simulink model "speedloop"  (R2021b)
settings: Solver=FixedStepAuto  StartTime=0.0  StopTime=10.0  FixedStep=1e-4  RelTol=1e-3
values from neighbouring files (symbols this model uses):
  CurrKi = 0.17    [speedloop.sldd]
  CurrKp = 35.0    [speedloop.sldd]
  flux = 0.016884    [speedloop.sldd]
  Pn = 4.0    [speedloop.sldd]
  SpeedKi = 0.0144    [speedloop.sldd]
  SpeedKp = 0.03389    [speedloop.sldd]
  Ubus = 24.0    [speedloop.sldd]
undefined symbols (not defined in the file or in its folder): DiscIntNeverNeededParam, sigbuilder_block
libraries: slpidlib x3, mcbplantlib x1, autolibpmsmexterior x1
settings Model: DataDictionary=speedloop.sldd  Creator=ssc  LastModifiedBy=ssc

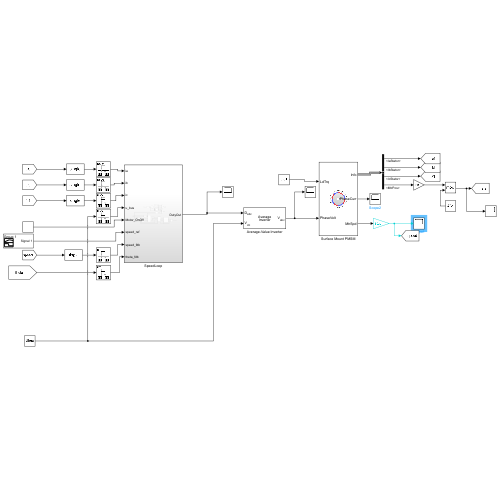
[thumbnail: Simulink's stored preview of the top-level diagram]
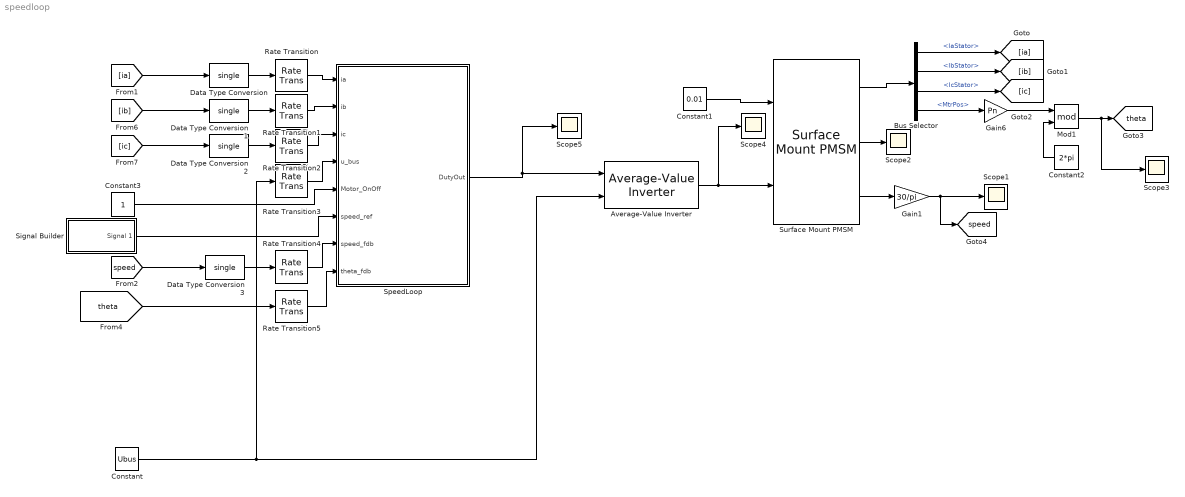
== system speedloop ==
  Average-Value Inverter : mcbplantlib/Average-Value Inverter
  Bus Selector : BusSelector  OutputSignals=IaStator,IbStator,IcStator,MtrPos
  Constant : Constant  Value=Ubus
  Constant1 : Constant  Value=0.01
  Constant2 : Constant  Value=2*pi  OutDataTypeStr=single
  Constant3 : Constant
  Data Type Conversion{,1..3} (4 alike) : DataTypeConversion  OutDataTypeStr=single
  Gain1 : Gain  Gain=30/pi  OutDataTypeStr=single
  Gain6 : Gain  Gain=Pn  OutDataTypeStr=single
  Mod1 : Math  Operator=mod  OutputSignalType=real  SaturateOnIntegerOverflow=on
  Rate Transition{,1..5} (6 alike) : RateTransition
  Scope{1..5} (5 alike) : Scope
  Signal Builder : Subsystem  Tag=STV Subsys  LoadFcn=sigbuilder_block('load');  StartFcn=sigbuilder_block('start');  StopFcn=sigbuilder_block('stop');  ClipboardFcn=sigbuilder_block('clipboard');  mask(Sigbuilder block){tuvar=[0:10]}
      mask help: Simulink:masks:SigbuilderBlock_MD
      mask init:
      | if ~strcmp(get_param(bdroot(gcbh),'SimulationStatus'),'stopped') tuvar = sigbuilder_block('maskInit'); end
      settings: CopyFcn=sigbuilder_block('copy');  DeleteFcn=sigbuilder_block('delete');  ModelCloseFcn=sigbuilder_block('modelClose');  PreSaveFcn=sigbuilder_block('preSave');  PauseFcn=sigbuilder_block('pause');  ContinueFcn=sigbuilder_block('continue');  NameChangeFcn=sigbuilder_block('namechange');  OpenFcn=sigbuilder_block('open',[367.2 103.2 550.8 400.2 ]);  CloseFcn=sigbuilder_block('close');
      mask Display: plot(0, 0, 100, 100,[2, 2, 32, 32, 2], [68, 8, 8, 68, 68],[32, 2], [38, 38], [32, 19, 2],[53, 60, 44], [32, 17, 17, 2],[16, 16, 31, 31]);txt = getActiveGroup(gcbh);text(2, 100, txt,'verticalAlignment', 'top');
  SpeedLoop : Subsystem
  Surface Mount PMSM : autolibpmsmexterior/Surface Mount PMSM  port_config=Torque  sim_type=Continuous  Ts=0.001  P=Pn  Rs=Rs  Ldq_=L  KConstText=Permanent flux linkage constant (lambda_pm):  lambda_pm=flux  Ke=159.9771  Kt=1.323  mechanical=[75e-6,8e-5,0]  idq0=[0 0]  theta_init=0  omega_init=0  KConst=flux  lambda_pm_calc=flux  RefBlkName='autolibpmsmexterior/Surface Mount PMSM'  aMode=5  Ldq="[0.0017      0.0017]"
      settings: SourceProductBaseCode=PW,DR,MT,UV,VE
  tag scope: speed=global, theta=global
  wires:
  SpeedLoop/1(DutyOut) -> Scope5/1, Average-Value Inverter/1
  Surface Mount PMSM/3 -> Gain1/1
  Surface Mount PMSM/1 -> Bus Selector/1
  Constant1/1 -> Surface Mount PMSM/1
  Bus Selector/1 -> [ia]  "<IaStator>"
  Gain1/1 -> Scope1/1, [speed]
  Surface Mount PMSM/2 -> Scope2/1
  Gain6/1 -> Mod1/1
  Bus Selector/2 -> [ib]  "<IbStator>"
  Mod1/1 -> Scope3/1, [theta]
  Constant2/1 -> Mod1/2
  Bus Selector/4 -> Gain6/1  "<MtrPos>"
  Constant/1 -> Rate Transition3/1, Average-Value Inverter/2
  Average-Value Inverter/1 -> Scope4/1, Surface Mount PMSM/2
  Bus Selector/3 -> [ic]  "<IcStator>"
  Data Type Conversion/1 -> Rate Transition/1
  Data Type Conversion1/1 -> Rate Transition1/1
  [ic] -> Data Type Conversion2/1
  [ib] -> Data Type Conversion1/1
  [ia] -> Data Type Conversion/1
  Data Type Conversion2/1 -> Rate Transition2/1
  Rate Transition/1 -> SpeedLoop/1(ia)
  Rate Transition1/1 -> SpeedLoop/2(ib)
  Rate Transition2/1 -> SpeedLoop/3(ic)
  Rate Transition3/1 -> SpeedLoop/4(u_bus)
  Constant3/1 -> SpeedLoop/5(Motor_OnOff)
  [speed] -> Data Type Conversion3/1
  Rate Transition4/1 -> SpeedLoop/7(speed_fdb)
  Data Type Conversion3/1 -> Rate Transition4/1
  Signal Builder/1(Signal 1) -> SpeedLoop/6(speed_ref)
  [theta] -> Rate Transition5/1
  Rate Transition5/1 -> SpeedLoop/8(theta_fdb)

== system speedloop/Signal Builder ==
  Demux : Demux  Tag=STV Demux  Outputs=1
      settings: DisplayOption=none
  FromWs : FromWorkspace  Tag=STV FromWs  VariableName=tuvar
      SigBuilderData=|
      | common.afterFinalStr = 'Extrapolate'
      | common.sampleTime = 0
      | dataSet.timeRange = [0 10]
      | dataSet.name = 'Group 1'
      | sbobj.Groups.Name = 'Group 1'
      | sbobj.Groups.Signals.Name = 'Signal 1'
      | sbobj.Groups.Signals.XData = [0 4 4 6 6 10]
      | sbobj.Groups.Signals.YData = [800 800 1000 1000 1200 1200]
  Signal 1 : Outport  Tag=STV Outport
  wires:
  Demux/1 -> Signal 1/1
  FromWs/1 -> Demux/1

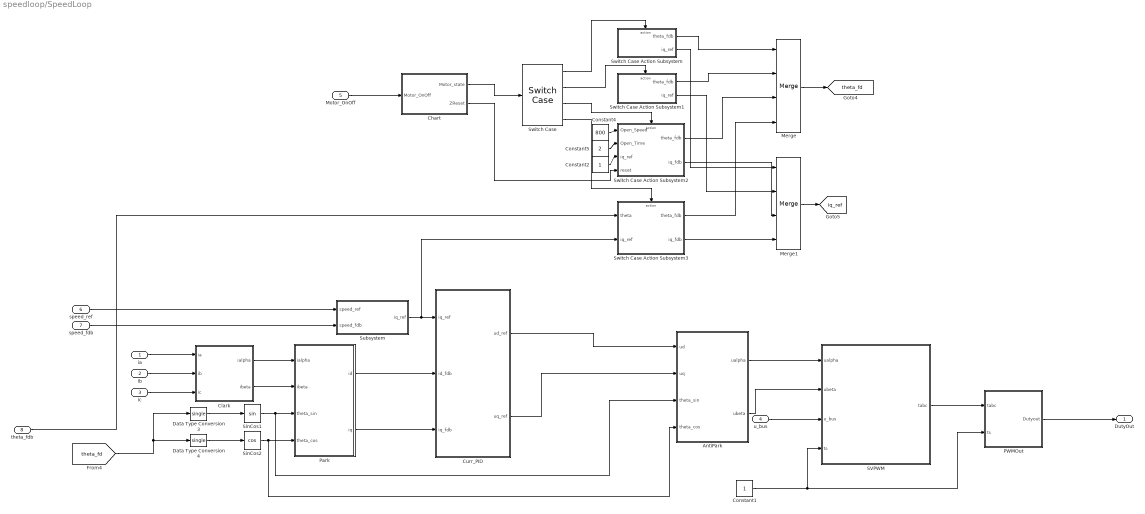
== system speedloop/SpeedLoop ==
  ia : Inport
  ib : Inport  Port=2
  ic : Inport  Port=3
  u_bus : Inport  Port=4
  Motor_OnOff : Inport  Port=5
  speed_ref : Inport  Port=6
  speed_fdb : Inport  Port=7
  theta_fdb : Inport  Port=8
  AntiPark : Subsystem
  Chart : Stateflow chart  TreatAsAtomicUnit=on
  Clark : Subsystem
  Constant1 : Constant
  Constant2 : Constant
  Constant4 : Constant  Value=800
  Constant5 : Constant  Value=2
  Curr_PID : Subsystem
  Data Type Conversion3 : DataTypeConversion  OutDataTypeStr=single
  Data Type Conversion4 : DataTypeConversion  OutDataTypeStr=single
  Merge : Merge  Inputs=4
  Merge1 : Merge  Inputs=4
  PWMOut : Subsystem
  Park : Subsystem
  SVPWM : Subsystem
  SinCos1 : Trigonometry
  SinCos2 : Trigonometry  Operator=cos
  Subsystem : Subsystem
  Switch Case : SwitchCase  CaseConditions={1,2,3,4}  ShowDefaultCase=off
  Switch Case Action Subsystem : Subsystem  TreatAsAtomicUnit=on
  Switch Case Action Subsystem1 : Subsystem  TreatAsAtomicUnit=on
  Switch Case Action Subsystem2 : Subsystem  TreatAsAtomicUnit=on
  Switch Case Action Subsystem3 : Subsystem  TreatAsAtomicUnit=on
  DutyOut : Outport
  tag scope: iq_ref=global, theta_fd=global
  wires:
  SinCos1/1 -> AntiPark/3(theta_sin), Park/3(theta_sin)
  Constant1/1 -> PWMOut/2(ts), SVPWM/4(ts)
  Switch Case Action Subsystem2/2(iq_fdb) -> Merge1/3
  Park/2(iq) -> Curr_PID/3(iq_fdb)
  Merge1/1 -> [iq_ref]
  Switch Case Action Subsystem/1(theta_fdb) -> Merge/1
  Switch Case Action Subsystem3/2(iq_fdb) -> Merge1/4
  Constant5/1 -> Switch Case Action Subsystem2/2(Open_Time)
  PWMOut/1(Dutyout) -> DutyOut/1
  SVPWM/1(tabc) -> PWMOut/1(tabc)
  Merge/1 -> [theta_fd]
  AntiPark/2(ubeta) -> SVPWM/2(ubeta)
  Chart/1(Motor_state) -> Switch Case/1
  ia/1 -> Clark/1(ia)
  Switch Case/4 -> Switch Case Action Subsystem3/Action
  theta_fdb/1 -> Switch Case Action Subsystem3/1(theta)
  Constant4/1 -> Switch Case Action Subsystem2/1(Open_Speed)
  Curr_PID/2(uq_ref) -> AntiPark/2(uq)
  Data Type Conversion3/1 -> SinCos1/1
  Switch Case Action Subsystem2/1(theta_fdb) -> Merge/3
  Switch Case Action Subsystem1/1(theta_fdb) -> Merge/2
  Clark/2(ibeta) -> Park/2(ibeta)
  Switch Case Action Subsystem1/2(iq_ref) -> Merge1/2
  u_bus/1 -> SVPWM/3(u_bus)
  Clark/1(ialpha) -> Park/1(ialpha)
  SinCos2/1 -> AntiPark/4(theta_cos), Park/4(theta_cos)
  Switch Case/1 -> Switch Case Action Subsystem/Action
  AntiPark/1(ualpha) -> SVPWM/1(ualpha)
  Switch Case/3 -> Switch Case Action Subsystem2/Action
  Park/1(id) -> Curr_PID/2(id_fdb)
  Switch Case/2 -> Switch Case Action Subsystem1/Action
  Data Type Conversion4/1 -> SinCos2/1
  ib/1 -> Clark/2(ib)
  Switch Case Action Subsystem/2(iq_ref) -> Merge1/1
  Curr_PID/1(ud_ref) -> AntiPark/1(ud)
  ic/1 -> Clark/3(ic)
  Motor_OnOff/1 -> Chart/1(Motor_OnOff)
  speed_ref/1 -> Subsystem/1(speed_ref)
  speed_fdb/1 -> Subsystem/2(speed_fdb)
  Constant2/1 -> Switch Case Action Subsystem2/3(iq_ref)
  Chart/2(ZReset) -> Switch Case Action Subsystem2/4(reset)
  [theta_fd] -> Data Type Conversion4/1, Data Type Conversion3/1
  Subsystem/1(iq_ref) -> Switch Case Action Subsystem3/2(iq_ref), Curr_PID/1(iq_ref)
  Switch Case Action Subsystem3/1(theta_fdb) -> Merge/4

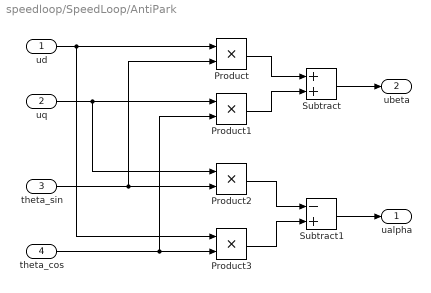
== system speedloop/SpeedLoop/AntiPark ==
  ud : Inport
  uq : Inport  Port=2
  theta_sin : Inport  Port=3
  theta_cos : Inport  Port=4
  Product{,1..3} (4 alike) : Product
  Subtract : Sum
  Subtract1 : Sum  Inputs=-+
  ualpha : Outport
  ubeta : Outport  Port=2
  wires:
  ud/1 -> Product/1, Product3/1
  theta_sin/1 -> Product2/2, Product/2
  uq/1 -> Product1/1, Product2/1
  theta_cos/1 -> Product3/2, Product1/2
  Product/1 -> Subtract/1
  Product1/1 -> Subtract/2
  Product2/1 -> Subtract1/1
  Product3/1 -> Subtract1/2
  Subtract/1 -> ubeta/1
  Subtract1/1 -> ualpha/1

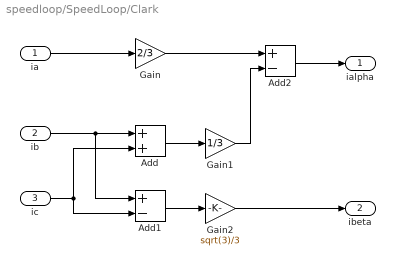
== system speedloop/SpeedLoop/Clark ==
  ia : Inport
  ib : Inport  Port=2
  ic : Inport  Port=3
  Add : Sum
  Add1 : Sum  Inputs=+-
  Add2 : Sum  Inputs=+-
  Gain : Gain  Gain=2/3
  Gain1 : Gain  Gain=1/3
  Gain2 : Gain  Gain=sqrt(3)/3
  ialpha : Outport
  ibeta : Outport  Port=2
  wires:
  ia/1 -> Gain/1
  ib/1 -> Add1/1, Add/1
  ic/1 -> Add1/2, Add/2
  Add/1 -> Gain1/1
  Add1/1 -> Gain2/1
  Gain1/1 -> Add2/2
  Gain/1 -> Add2/1
  Gain2/1 -> ibeta/1
  Add2/1 -> ialpha/1

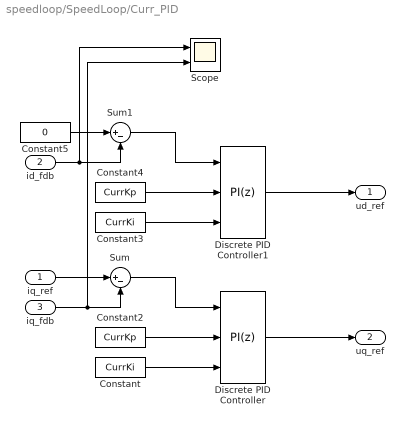
== system speedloop/SpeedLoop/Curr_PID ==
  iq_ref : Inport
  id_fdb : Inport  Port=2
  iq_fdb : Inport  Port=3
  Constant : Constant  Value=CurrKi
  Constant2 : Constant  Value=CurrKp
  Constant3 : Constant  Value=CurrKi
  Constant4 : Constant  Value=CurrKp
  Constant5 : Constant  Value=0
  Discrete PID Controller : slpidlib/PID Controller  Controller=PI  Form=Parallel  TimeDomain=Discrete-time  UseExternalTs=off  SampleTime=-1  IntegratorMethod=Forward Euler  FilterMethod=Forward Euler  ControllerParametersSource=external  P=1  I=1  D=0  UseFilter=on  N=100  TunerSelectOption=Transfer Function Based (PID Tuner App)  InitialConditionSource=internal  InitialConditionForIntegrator=0  InitialConditionForFilter=0  DifferentiatorICPrevScaledInput=0  ExternalReset=none  TrackingMode=off  Kt=1  LimitOutput=on  SatLimitsSource=internal  UpperSaturationLimit=Ubus/sqrt(3)  LowerSaturationLimit=-Ubus/sqrt(3)  LinearizeAsGain=off  AntiWindupMode=clamping  Kb=1  POutMin=[]  POutMax=[]  IOutMin=[]  IOutMax=[]  DOutMin=[]  DOutMax=[]  NOutMin=[]  NOutMax=[]  SumOutMin=[]  SumOutMax=[]  SaturationOutMin=[]  SaturationOutMax=[]  PParamMin=[]  PParamMax=[]  IParamMin=[]  IParamMax=[]  DParamMin=[]  DParamMax=[]  NParamMin=[]  NParamMax=[]  KbParamMin=[]  KbParamMax=[]  KtParamMin=[]  KtParamMax=[]  KbOutMin=[]  KbOutMax=[]  KtOutMin=[]  KtOutMax=[]  IntegratorOutMin=[]  IntegratorOutMax=[]  FilterOutMin=[]  FilterOutMax=[]  SumI1OutMin=[]  SumI1OutMax=[]  SumI2OutMin=[]  SumI2OutMax=[]  SumI3OutMin=[]  SumI3OutMax=[]  SumI4OutMin=[]  SumI4OutMax=[]  SumDOutMin=[]  SumDOutMax=[]  DifferentiatorOutMin=[]  DifferentiatorOutMax=[]  FilterDiffOutCoefMin=[]  FilterDiffOutCoefMax=[]  ReciprocalOutMin=[]  ReciprocalOutMax=[]  SumDenOutMin=[]  SumDenOutMax=[]  SumNumOutMin=[]  SumNumOutMax=[]  DivideOutMin=[]  DivideOutMax=[]  UdiffTsProdOutMin=[]  UdiffTsProdOutMax=[]  NTsProdOutMin=[]  NTsProdOutMax=[]  UintegralTsProdOutMin=[]  UintegralTsProdOutMax=[]  UngainTsProdOutMin=[]  UngainTsProdOutMax=[]  IntegratorContinuousStateAttributes=''  IntegratorStateMustResolveToSignalObject=off  IntegratorRTWStateStorageClass=Auto  FilterContinuousStateAttributes=''  FilterStateMustResolveToSignalObject=off  FilterRTWStateStorageClass=Auto  ParallelPVariant=ExternalParameters  IdealPVariant=Disabled  IVariant=ExternalParameters  DVariant=Disabled  IntegratorVariant=Discrete  SatVariant=Enabled  AWVariant=DiscClampingParallel  PCopyVariant=Disabled  TRVariant=Disabled  FdbkBlocksVariant=Forward  IdealPFdbkVariant=Disabled  SatFdbkVariant=Disabled  DerivativeFilterVariant=Disabled  NVariant=Disabled  NCopyVariant=Disabled_SignalSpec  FilterICVariant=Disabled  IntegratorICVariant=InternalICs  ExternalResetVariant=Disabled  TRSumVariant=Passthrough  SumFdbkVariant=Disabled  SumVariant=Sum_PI  TsampFilterVariant=InternalTs  TsampNgainVariant=Passthrough  TsampIntegralVariant=Passthrough  ExternalSaturationOutDataTypeStr=Inherit: Same as second input
  Discrete PID Controller1 : slpidlib/PID Controller  Controller=PI  Form=Parallel  TimeDomain=Discrete-time  UseExternalTs=off  SampleTime=-1  IntegratorMethod=Forward Euler  FilterMethod=Forward Euler  ControllerParametersSource=external  P=1  I=1  D=0  UseFilter=on  N=100  TunerSelectOption=Transfer Function Based (PID Tuner App)  InitialConditionSource=internal  InitialConditionForIntegrator=0  InitialConditionForFilter=0  DifferentiatorICPrevScaledInput=0  ExternalReset=none  TrackingMode=off  Kt=1  LimitOutput=on  SatLimitsSource=internal  UpperSaturationLimit=Ubus/sqrt(3)  LowerSaturationLimit=-Ubus/sqrt(3)  LinearizeAsGain=off  AntiWindupMode=clamping  Kb=1  POutMin=[]  POutMax=[]  IOutMin=[]  IOutMax=[]  DOutMin=[]  DOutMax=[]  NOutMin=[]  NOutMax=[]  SumOutMin=[]  SumOutMax=[]  SaturationOutMin=[]  SaturationOutMax=[]  PParamMin=[]  PParamMax=[]  IParamMin=[]  IParamMax=[]  DParamMin=[]  DParamMax=[]  NParamMin=[]  NParamMax=[]  KbParamMin=[]  KbParamMax=[]  KtParamMin=[]  KtParamMax=[]  KbOutMin=[]  KbOutMax=[]  KtOutMin=[]  KtOutMax=[]  IntegratorOutMin=[]  IntegratorOutMax=[]  FilterOutMin=[]  FilterOutMax=[]  SumI1OutMin=[]  SumI1OutMax=[]  SumI2OutMin=[]  SumI2OutMax=[]  SumI3OutMin=[]  SumI3OutMax=[]  SumI4OutMin=[]  SumI4OutMax=[]  SumDOutMin=[]  SumDOutMax=[]  DifferentiatorOutMin=[]  DifferentiatorOutMax=[]  FilterDiffOutCoefMin=[]  FilterDiffOutCoefMax=[]  ReciprocalOutMin=[]  ReciprocalOutMax=[]  SumDenOutMin=[]  SumDenOutMax=[]  SumNumOutMin=[]  SumNumOutMax=[]  DivideOutMin=[]  DivideOutMax=[]  UdiffTsProdOutMin=[]  UdiffTsProdOutMax=[]  NTsProdOutMin=[]  NTsProdOutMax=[]  UintegralTsProdOutMin=[]  UintegralTsProdOutMax=[]  UngainTsProdOutMin=[]  UngainTsProdOutMax=[]  IntegratorContinuousStateAttributes=''  IntegratorStateMustResolveToSignalObject=off  IntegratorRTWStateStorageClass=Auto  FilterContinuousStateAttributes=''  FilterStateMustResolveToSignalObject=off  FilterRTWStateStorageClass=Auto  ParallelPVariant=ExternalParameters  IdealPVariant=Disabled  IVariant=ExternalParameters  DVariant=Disabled  IntegratorVariant=Discrete  SatVariant=Enabled  AWVariant=DiscClampingParallel  PCopyVariant=Disabled  TRVariant=Disabled  FdbkBlocksVariant=Forward  IdealPFdbkVariant=Disabled  SatFdbkVariant=Disabled  DerivativeFilterVariant=Disabled  NVariant=Disabled  NCopyVariant=Disabled_SignalSpec  FilterICVariant=Disabled  IntegratorICVariant=InternalICs  ExternalResetVariant=Disabled  TRSumVariant=Passthrough  SumFdbkVariant=Disabled  SumVariant=Sum_PI  TsampFilterVariant=InternalTs  TsampNgainVariant=Passthrough  TsampIntegralVariant=Passthrough  ExternalSaturationOutDataTypeStr=Inherit: Same as second input
  Scope : Scope  NumInputPorts=2
  Sum : Sum  Inputs=|+-
  Sum1 : Sum  Inputs=|+-
  ud_ref : Outport
  uq_ref : Outport  Port=2
  wires:
  Constant2/1 -> Discrete PID Controller/2
  Constant3/1 -> Discrete PID Controller1/3
  Sum1/1 -> Discrete PID Controller1/1
  Sum/1 -> Discrete PID Controller/1
  Constant/1 -> Discrete PID Controller/3
  iq_ref/1 -> Sum/1
  Discrete PID Controller/1 -> uq_ref/1
  Constant4/1 -> Discrete PID Controller1/2
  Discrete PID Controller1/1 -> ud_ref/1
  Constant5/1 -> Sum1/1
  iq_fdb/1 -> Scope/2, Sum/2
  id_fdb/1 -> Scope/1, Sum1/2

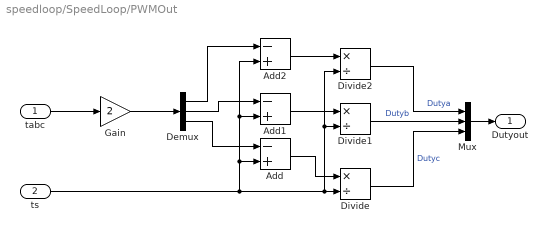
== system speedloop/SpeedLoop/PWMOut ==
  tabc : Inport
  ts : Inport  Port=2
  Add : Sum  Inputs=-+
  Add1 : Sum  Inputs=-+
  Add2 : Sum  Inputs=-+
  Demux : Demux  Outputs=3
  Divide : Product  Inputs=*/
  Divide1 : Product  Inputs=*/
  Divide2 : Product  Inputs=*/
  Gain : Gain  Gain=2
  Mux : Mux  Inputs=3
  Dutyout : Outport
  wires:
  tabc/1 -> Gain/1
  Gain/1 -> Demux/1
  ts/1 -> Add1/2, Add2/2, Add/2, Divide2/2, Divide1/2, Divide/2
  Demux/3 -> Add/1
  Add/1 -> Divide/1
  Divide/1 -> Mux/3  "Dutyc"
  Demux/1 -> Add2/1
  Add1/1 -> Divide1/1
  Add2/1 -> Divide2/1
  Demux/2 -> Add1/1
  Divide1/1 -> Mux/2  "Dutyb"
  Divide2/1 -> Mux/1  "Dutya"
  Mux/1 -> Dutyout/1

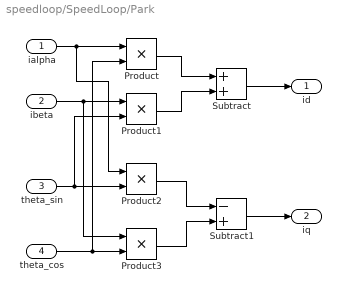
== system speedloop/SpeedLoop/Park ==
  ialpha : Inport
  ibeta : Inport  Port=2
  theta_sin : Inport  Port=3
  theta_cos : Inport  Port=4
  Product{,1..3} (4 alike) : Product
  Subtract : Sum
  Subtract1 : Sum  Inputs=-+
  id : Outport
  iq : Outport  Port=2
  wires:
  ialpha/1 -> Product2/1, Product/1
  theta_cos/1 -> Product/2, Product3/2
  ibeta/1 -> Product3/1, Product1/1
  theta_sin/1 -> Product1/2, Product2/2
  Product/1 -> Subtract/1
  Product1/1 -> Subtract/2
  Subtract/1 -> id/1
  Product2/1 -> Subtract1/1
  Product3/1 -> Subtract1/2
  Subtract1/1 -> iq/1

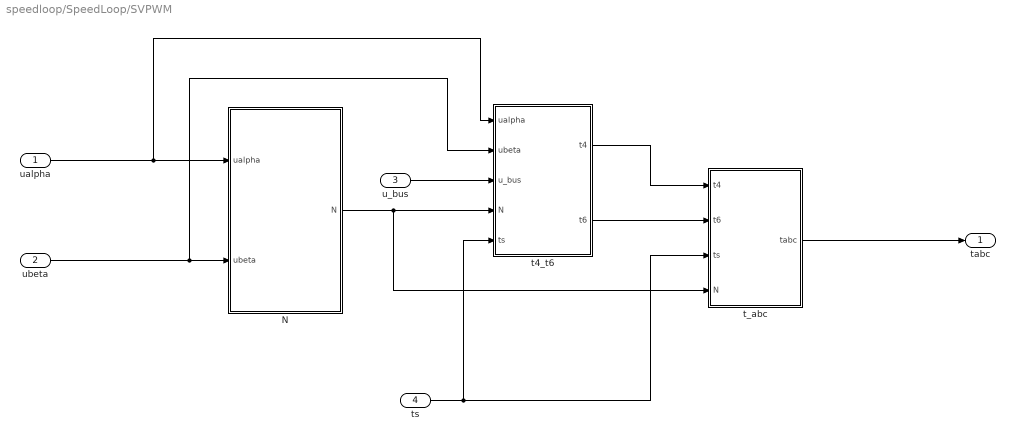
== system speedloop/SpeedLoop/SVPWM ==
  ualpha : Inport
  ubeta : Inport  Port=2
  u_bus : Inport  Port=3
  ts : Inport  Port=4
  N : Subsystem
  t4_t6 : Subsystem
  t_abc : Subsystem
  tabc : Outport
  wires:
  ubeta/1 -> t4_t6/2(ubeta), N/2(ubeta)
  t4_t6/1(t4) -> t_abc/1(t4)
  N/1(N) -> t_abc/4(N), t4_t6/4(N)
  ualpha/1 -> t4_t6/1(ualpha), N/1(ualpha)
  t4_t6/2(t6) -> t_abc/2(t6)
  u_bus/1 -> t4_t6/3(u_bus)
  ts/1 -> t_abc/3(ts), t4_t6/5(ts)
  t_abc/1(tabc) -> tabc/1

== system speedloop/SpeedLoop/Subsystem ==
  speed_ref : Inport
  speed_fdb : Inport  Port=2
  Constant2 : Constant  Value=SpeedKp
  Constant3 : Constant  Value=SpeedKi
  Discrete PID Controller1 : slpidlib/PID Controller  Controller=PI  Form=Parallel  TimeDomain=Discrete-time  UseExternalTs=off  SampleTime=-1  IntegratorMethod=Forward Euler  FilterMethod=Forward Euler  ControllerParametersSource=external  P=1  I=1  D=0  UseFilter=on  N=100  TunerSelectOption=Transfer Function Based (PID Tuner App)  InitialConditionSource=internal  InitialConditionForIntegrator=0  InitialConditionForFilter=0  DifferentiatorICPrevScaledInput=0  ExternalReset=none  TrackingMode=off  Kt=1  LimitOutput=on  SatLimitsSource=internal  UpperSaturationLimit=3  LowerSaturationLimit=-3  LinearizeAsGain=off  AntiWindupMode=clamping  Kb=1  POutMin=[]  POutMax=[]  IOutMin=[]  IOutMax=[]  DOutMin=[]  DOutMax=[]  NOutMin=[]  NOutMax=[]  SumOutMin=[]  SumOutMax=[]  SaturationOutMin=[]  SaturationOutMax=[]  PParamMin=[]  PParamMax=[]  IParamMin=[]  IParamMax=[]  DParamMin=[]  DParamMax=[]  NParamMin=[]  NParamMax=[]  KbParamMin=[]  KbParamMax=[]  KtParamMin=[]  KtParamMax=[]  KbOutMin=[]  KbOutMax=[]  KtOutMin=[]  KtOutMax=[]  IntegratorOutMin=[]  IntegratorOutMax=[]  FilterOutMin=[]  FilterOutMax=[]  SumI1OutMin=[]  SumI1OutMax=[]  SumI2OutMin=[]  SumI2OutMax=[]  SumI3OutMin=[]  SumI3OutMax=[]  SumI4OutMin=[]  SumI4OutMax=[]  SumDOutMin=[]  SumDOutMax=[]  DifferentiatorOutMin=[]  DifferentiatorOutMax=[]  FilterDiffOutCoefMin=[]  FilterDiffOutCoefMax=[]  ReciprocalOutMin=[]  ReciprocalOutMax=[]  SumDenOutMin=[]  SumDenOutMax=[]  SumNumOutMin=[]  SumNumOutMax=[]  DivideOutMin=[]  DivideOutMax=[]  UdiffTsProdOutMin=[]  UdiffTsProdOutMax=[]  NTsProdOutMin=[]  NTsProdOutMax=[]  UintegralTsProdOutMin=[]  UintegralTsProdOutMax=[]  UngainTsProdOutMin=[]  UngainTsProdOutMax=[]  IntegratorContinuousStateAttributes=''  IntegratorStateMustResolveToSignalObject=off  IntegratorRTWStateStorageClass=Auto  FilterContinuousStateAttributes=''  FilterStateMustResolveToSignalObject=off  FilterRTWStateStorageClass=Auto  ParallelPVariant=ExternalParameters  IdealPVariant=Disabled  IVariant=ExternalParameters  DVariant=Disabled  IntegratorVariant=Discrete  SatVariant=Enabled  AWVariant=DiscClampingParallel  PCopyVariant=Disabled  TRVariant=Disabled  FdbkBlocksVariant=Forward  IdealPFdbkVariant=Disabled  SatFdbkVariant=Disabled  DerivativeFilterVariant=Disabled  NVariant=Disabled  NCopyVariant=Disabled_SignalSpec  FilterICVariant=Disabled  IntegratorICVariant=InternalICs  ExternalResetVariant=Disabled  TRSumVariant=Passthrough  SumFdbkVariant=Disabled  SumVariant=Sum_PI  TsampFilterVariant=InternalTs  TsampNgainVariant=Passthrough  TsampIntegralVariant=Passthrough  ExternalSaturationOutDataTypeStr=Inherit: Same as second input
  Sum1 : Sum  Inputs=|+-
  iq_ref : Outport
  wires:
  speed_fdb/1 -> Sum1/2
  Constant2/1 -> Discrete PID Controller1/2
  speed_ref/1 -> Sum1/1
  Discrete PID Controller1/1 -> iq_ref/1
  Sum1/1 -> Discrete PID Controller1/1
  Constant3/1 -> Discrete PID Controller1/3

== system speedloop/SpeedLoop/Switch Case Action Subsystem ==
  Action Port : ActionPort  ActionPortLabel=case [ 1 ]:
  Constant : Constant  Value=0
  Constant1 : Constant  Value=0
  theta_fdb : Outport
  iq_ref : Outport  Port=2
  wires:
  Constant/1 -> theta_fdb/1
  Constant1/1 -> iq_ref/1

== system speedloop/SpeedLoop/Switch Case Action Subsystem1 ==
  Action Port : ActionPort  ActionPortLabel=case [ 2 ]:
  Constant : Constant  Value=0
  Constant1 : Constant
  theta_fdb : Outport
  iq_ref : Outport  Port=2
  wires:
  Constant/1 -> theta_fdb/1
  Constant1/1 -> iq_ref/1

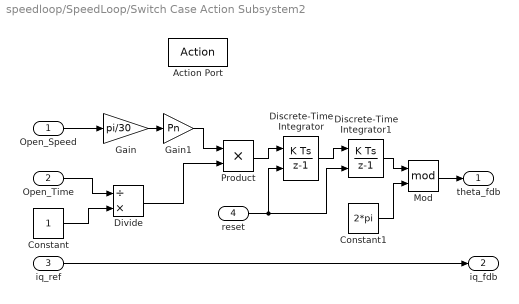
== system speedloop/SpeedLoop/Switch Case Action Subsystem2 ==
  Open_Speed : Inport
  Open_Time : Inport  Port=2
  iq_ref : Inport  Port=3
  reset : Inport  Port=4
  Action Port : ActionPort  ActionPortLabel=case [ 3 ]:
  Constant : Constant
  Constant1 : Constant  Value=2*pi  OutDataTypeStr=double
  Discrete-Time Integrator : DiscreteIntegrator  ExternalReset=rising  SampleTime=-1  ICPrevOutput=DiscIntNeverNeededParam  ICPrevScaledInput=DiscIntNeverNeededParam
  Discrete-Time Integrator1 : DiscreteIntegrator  ExternalReset=rising  SampleTime=-1  ICPrevOutput=DiscIntNeverNeededParam  ICPrevScaledInput=DiscIntNeverNeededParam
  Divide : Product  Inputs=/*
  Gain : Gain  Gain=pi/30
  Gain1 : Gain  Gain=Pn
  Mod : Math  Operator=mod  SaturateOnIntegerOverflow=on
  Product : Product
  theta_fdb : Outport
  iq_fdb : Outport  Port=2
  wires:
  Open_Speed/1 -> Gain/1
  Gain/1 -> Gain1/1
  Gain1/1 -> Product/1
  Open_Time/1 -> Divide/1
  Constant/1 -> Divide/2
  Divide/1 -> Product/2
  Product/1 -> Discrete-Time Integrator/1
  iq_ref/1 -> iq_fdb/1
  Discrete-Time Integrator/1 -> Discrete-Time Integrator1/1
  Mod/1 -> theta_fdb/1
  Constant1/1 -> Mod/2
  Discrete-Time Integrator1/1 -> Mod/1
  reset/1 -> Discrete-Time Integrator/2, Discrete-Time Integrator1/2

== system speedloop/SpeedLoop/Switch Case Action Subsystem3 ==
  theta : Inport
  iq_ref : Inport  Port=2
  Action Port : ActionPort  ActionPortLabel=case [ 4 ]:
  Data Type Conversion1 : DataTypeConversion  OutDataTypeStr=double
  theta_fdb : Outport
  iq_fdb : Outport  Port=2
  wires:
  iq_ref/1 -> iq_fdb/1
  theta/1 -> Data Type Conversion1/1
  Data Type Conversion1/1 -> theta_fdb/1

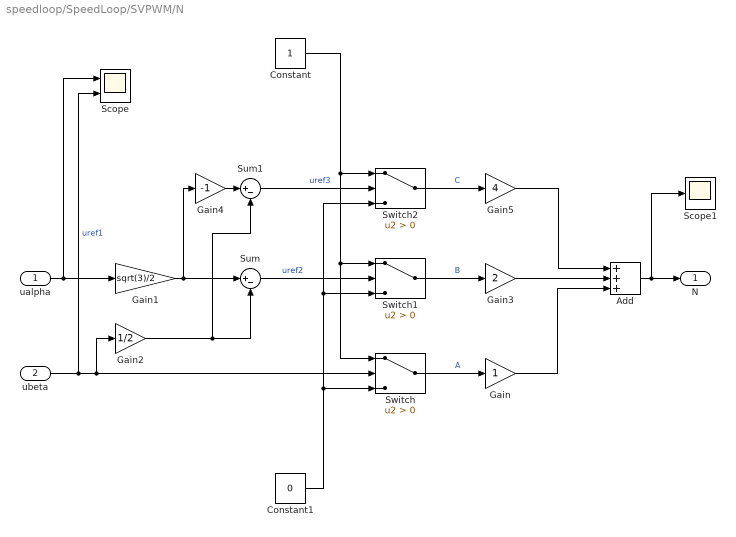
== system speedloop/SpeedLoop/SVPWM/N ==
  ualpha : Inport
  ubeta : Inport  Port=2
  Add : Sum  Inputs=+++
  Constant : Constant  OutDataTypeStr=single
  Constant1 : Constant  Value=0  OutDataTypeStr=single
  Gain : Gain
  Gain1 : Gain  Gain=sqrt(3)/2
  Gain2 : Gain  Gain=1/2
  Gain3 : Gain  Gain=2
  Gain4 : Gain  Gain=-1
  Gain5 : Gain  Gain=4
  Scope : Scope  NumInputPorts=2
  Scope1 : Scope
  Sum : Sum  Inputs=|+-
  Sum1 : Sum  Inputs=|+-
  Switch : Switch  Criteria=u2 > Threshold
  Switch1 : Switch  Criteria=u2 > Threshold
  Switch2 : Switch  Criteria=u2 > Threshold
  N : Outport
  wires:
  ualpha/1 -> Gain1/1, Scope/1
  ubeta/1 -> Switch/2, Gain2/1, Scope/2  "uref1"
  Constant/1 -> Switch2/1, Switch1/1, Switch/1
  Constant1/1 -> Switch2/3, Switch1/3, Switch/3
  Switch/1 -> Gain/1  "A"
  Gain1/1 -> Gain4/1, Sum/1
  Gain2/1 -> Sum1/2, Sum/2
  Sum/1 -> Switch1/2  "uref2"
  Switch1/1 -> Gain3/1  "B"
  Gain4/1 -> Sum1/1
  Sum1/1 -> Switch2/2  "uref3"
  Switch2/1 -> Gain5/1  "C"
  Gain3/1 -> Add/2
  Add/1 -> Scope1/1, N/1
  Gain/1 -> Add/3
  Gain5/1 -> Add/1

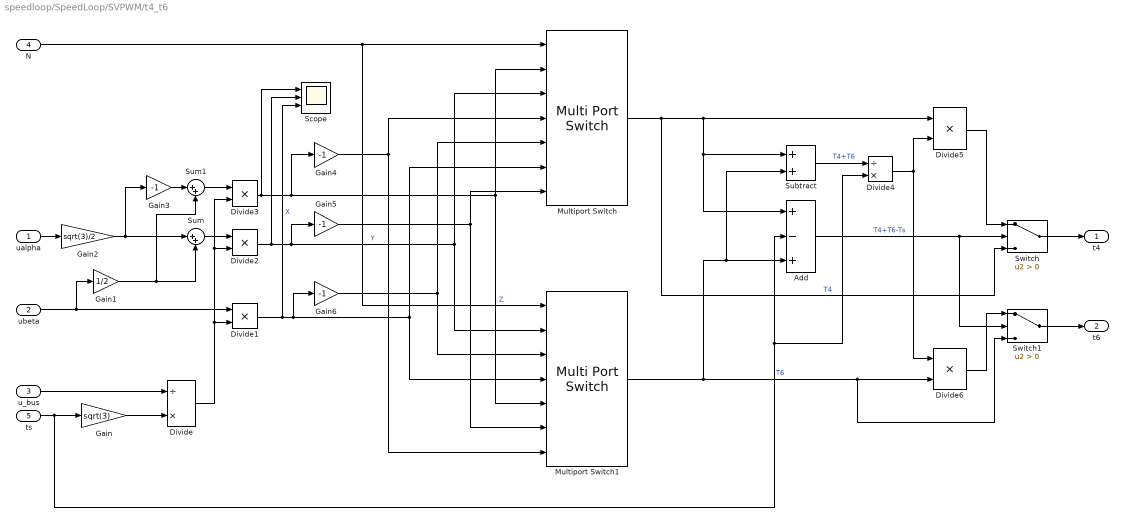
== system speedloop/SpeedLoop/SVPWM/t4_t6 ==
  ualpha : Inport
  ubeta : Inport  Port=2
  u_bus : Inport  Port=3
  N : Inport  Port=4
  ts : Inport  Port=5
  Add : Sum  Inputs=+-+
  Divide : Product  Inputs=/*
  Divide{1..3,5..6} (5 alike) : Product  Inputs=**
  Divide4 : Product  Inputs=/*
  Gain : Gain  Gain=sqrt(3)
  Gain1 : Gain  Gain=1/2
  Gain2 : Gain  Gain=sqrt(3)/2
  Gain{3..6} (4 alike) : Gain  Gain=-1
  Multiport Switch : MultiPortSwitch  Inputs=6  DiagnosticForDefault=None
  Multiport Switch1 : MultiPortSwitch  Inputs=6  DiagnosticForDefault=None
  Scope : Scope  NumInputPorts=3
  Subtract : Sum
  Sum : Sum  Inputs=|++
  Sum1 : Sum  Inputs=|++
  Switch : Switch  Criteria=u2 > Threshold
  Switch1 : Switch  Criteria=u2 > Threshold
  t4 : Outport
  t6 : Outport  Port=2
  wires:
  ts/1 -> Gain/1, Divide4/2, Add/2
  u_bus/1 -> Divide/1
  Gain/1 -> Divide/2
  ubeta/1 -> Gain1/1, Divide1/1
  Divide/1 -> Divide3/2, Divide2/2, Divide1/2
  Divide1/1 -> Scope/3, Multiport Switch1/4, Multiport Switch/6, Gain6/1  "X"
  ualpha/1 -> Gain2/1
  Gain1/1 -> Sum1/2, Sum/2
  Gain2/1 -> Gain3/1, Sum/1
  Sum/1 -> Divide2/1
  Divide2/1 -> Scope/2, Multiport Switch1/2, Multiport Switch/3, Gain5/1  "Y"
  Gain3/1 -> Sum1/1
  Sum1/1 -> Divide3/1
  Divide3/1 -> Scope/1, Gain4/1, Multiport Switch1/5, Multiport Switch/2  "Z"
  N/1 -> Multiport Switch1/1, Multiport Switch/1
  Multiport Switch/1 -> Switch/3, Divide5/1, Subtract/1, Add/1  "T4"
  Gain6/1 -> Multiport Switch1/3, Multiport Switch/5
  Gain4/1 -> Multiport Switch1/7, Multiport Switch/4
  Gain5/1 -> Multiport Switch1/6, Multiport Switch/7
  Add/1 -> Switch1/2, Switch/2  "T4+T6-Ts"
  Multiport Switch1/1 -> Switch1/3, Divide6/2, Subtract/2, Add/3  "T6"
  Subtract/1 -> Divide4/1  "T4+T6"
  Divide4/1 -> Divide5/2, Divide6/1
  Divide5/1 -> Switch/1
  Divide6/1 -> Switch1/1
  Switch/1 -> t4/1
  Switch1/1 -> t6/1

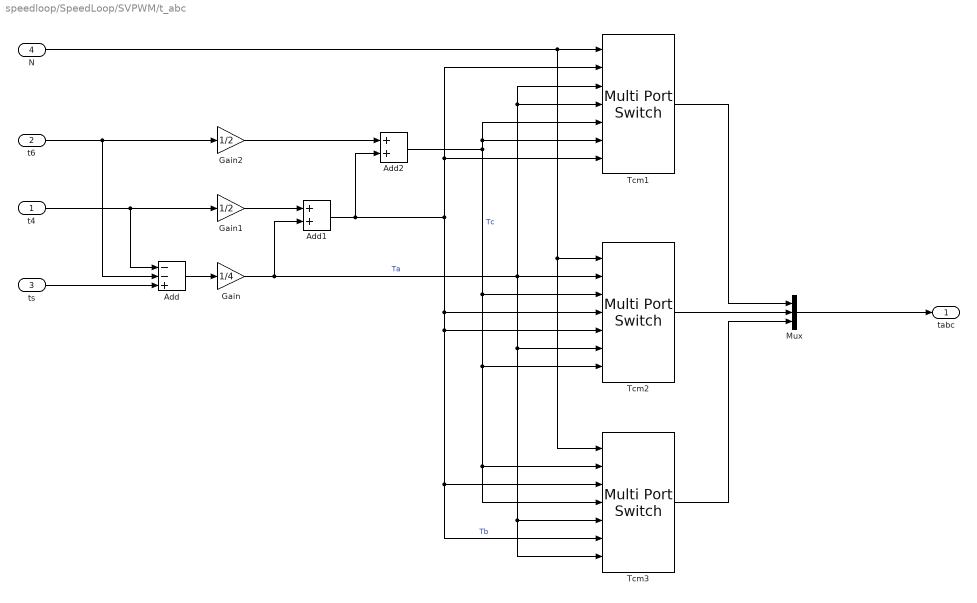
== system speedloop/SpeedLoop/SVPWM/t_abc ==
  t4 : Inport
  t6 : Inport  Port=2
  ts : Inport  Port=3
  N : Inport  Port=4
  Add : Sum  Inputs=--+
  Add1 : Sum
  Add2 : Sum
  Gain : Gain  Gain=1/4
  Gain1 : Gain  Gain=1/2
  Gain2 : Gain  Gain=1/2
  Mux : Mux  Inputs=3
  "Tcm1 " : MultiPortSwitch  Inputs=6  DiagnosticForDefault=None
  Tcm2 : MultiPortSwitch  Inputs=6  DiagnosticForDefault=None
  Tcm3 : MultiPortSwitch  Inputs=6  DiagnosticForDefault=None
  tabc : Outport
  wires:
  ts/1 -> Add/3
  t6/1 -> Add/2, Gain2/1
  t4/1 -> Add/1, Gain1/1
  Add/1 -> Gain/1
  Gain/1 -> Tcm2/6, Tcm3/7, Tcm3/5, "Tcm1 "/4, "Tcm1 "/3, Tcm2/2, Add1/2  "Ta"
  Gain1/1 -> Add1/1
  Gain2/1 -> Add2/1
  Add1/1 -> Add2/2, "Tcm1 "/7, "Tcm1 "/2, Tcm2/4, Tcm3/6, Tcm3/3, Tcm2/5  "Tb"
  N/1 -> Tcm3/1, Tcm2/1, "Tcm1 "/1
  Add2/1 -> "Tcm1 "/6, "Tcm1 "/5, Tcm3/4, Tcm3/2, Tcm2/7, Tcm2/3  "Tc"
  "Tcm1 "/1 -> Mux/1
  Tcm3/1 -> Mux/3
  Tcm2/1 -> Mux/2
  Mux/1 -> tabc/1

== stateflow chart speedloop/SpeedLoop/Chart ==
  state RunStage
    en:
    du:
    Motor_state = 4;
  state OpenStage
    en:
    ZReset = 0;
    cnt = 0;
    du:
    if cnt == 1
    ZReset = 1;
    end
    cnt = 1;
    Motor_state = 3;
  state AlignStage
    en:
    du:
    Motor_state = 2;
  state IDLE
    en:
    du:
    Motor_state = 1;
  (default) -> IDLE
  IDLE -> AlignStage : [Motor_OnOff ==1]
  AlignStage -> OpenStage [order 1] : [after(2000,tick)]
  OpenStage -> RunStage [order 2] : [after(20000,tick) ]
  AlignStage -> IDLE [order 2] : [Motor_OnOff == 0]
  RunStage -> IDLE : [Motor_OnOff ==0]
  OpenStage -> IDLE [order 1] : [Motor_OnOff ==0]
  data: Motor_OnOff input; Motor_state output; cnt local; ZReset output
